simulink model "VITM_OL_Harness"  (R2017b)
settings: Solver=ode4  StartTime=0.0  StopTime=sim_time  FixedStep=0.01  RelTol=1e-3  EnableMultiTasking=on
settings Model: Creator=favv5g  LastModifiedBy=nctzv8
settings DataIOCC: LimitDataPoints=on
settings OptimizationCC: LifeSpan=inf
settings DebuggingCC: MultiTaskRateTransMsg=warning  SingleTaskRateTransMsg=warning  AllowSymbolicDim=off  SFUnexpectedBacktrackingDiag=warning  SFNoUnconditionalDefaultTransitionDiag=warning  SFExecutionAtInitializationDiag=none
settings HardwareCC: ProdBitPerPointer=32  ProdBitPerSizeT=32  ProdBitPerPtrDiffT=32  ProdLargestAtomicInteger=Long  ProdLargestAtomicFloat=Double  ProdEndianess=BigEndian  ProdWordSize=32  ProdHWDeviceType=Freescale->32-bit PowerPC
settings ModelReferenceCC: PropagateSignalLabelsOutOfModel=off
settings CodeAppCC: StateflowObjectComments=on
settings GRTTargetCC: TargetLangStandard=C89/C90 (ANSI)
settings ConfigComp: CovMetricSettings=dw  CovHtmlReporting=on  CovSaveCumulativeToWorkspaceVar=on  CovSaveSingleToWorkspaceVar=on  CovExternalEMLEnable=off

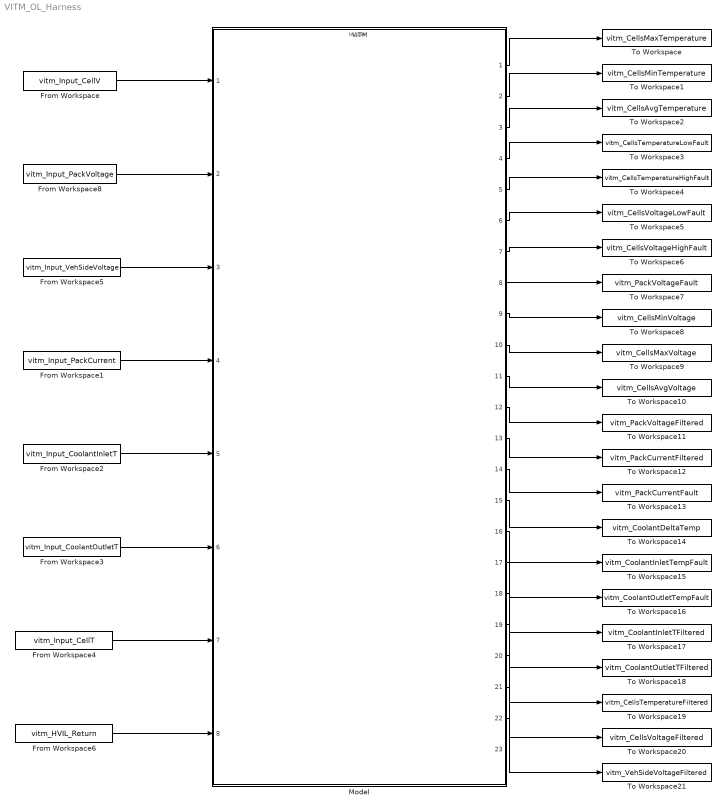
== system VITM_OL_Harness ==
  From Workspace : FromWorkspace  VariableName=vitm_Input_CellV  SampleTime=0
  From Workspace1 : FromWorkspace  VariableName=vitm_Input_PackCurrent  SampleTime=0
  From Workspace2 : FromWorkspace  VariableName=vitm_Input_CoolantInletT  SampleTime=0
  From Workspace3 : FromWorkspace  VariableName=vitm_Input_CoolantOutletT  SampleTime=0
  From Workspace4 : FromWorkspace  VariableName=vitm_Input_CellT  SampleTime=0
  From Workspace5 : FromWorkspace  VariableName=vitm_Input_VehSideVoltage  SampleTime=0
  From Workspace6 : FromWorkspace  VariableName=vitm_HVIL_Return  SampleTime=0
  From Workspace8 : FromWorkspace  VariableName=vitm_Input_PackVoltage  SampleTime=0
  Model : ModelReference  ModelNameDialog=VITM.slx  SimulationMode=Normal  ModelReferenceVersion=1.124  TriggerPortName=Trigger  TriggerPortTriggerType=function-call  TriggerPortStatesWhenEnabling=held
  To Workspace : ToWorkspace  VariableName=vitm_CellsMaxTemperature  SaveFormat=Timeseries  SampleTime=-1
  To Workspace1 : ToWorkspace  VariableName=vitm_CellsMinTemperature  SaveFormat=Timeseries  SampleTime=-1
  To Workspace10 : ToWorkspace  VariableName=vitm_CellsAvgVoltage  SaveFormat=Timeseries  SampleTime=-1
  To Workspace11 : ToWorkspace  VariableName=vitm_PackVoltageFiltered  SaveFormat=Timeseries  SampleTime=-1
  To Workspace12 : ToWorkspace  VariableName=vitm_PackCurrentFiltered  SaveFormat=Timeseries  SampleTime=-1
  To Workspace13 : ToWorkspace  VariableName=vitm_PackCurrentFault  SaveFormat=Timeseries  SampleTime=-1
  To Workspace14 : ToWorkspace  VariableName=vitm_CoolantDeltaTemp  SaveFormat=Timeseries  SampleTime=-1
  To Workspace15 : ToWorkspace  VariableName=vitm_CoolantInletTempFault  SaveFormat=Timeseries  SampleTime=-1
  To Workspace16 : ToWorkspace  VariableName=vitm_CoolantOutletTempFault  SaveFormat=Timeseries  SampleTime=-1
  To Workspace17 : ToWorkspace  VariableName=vitm_CoolantInletTFiltered  SaveFormat=Timeseries  SampleTime=-1
  To Workspace18 : ToWorkspace  VariableName=vitm_CoolantOutletTFiltered  SaveFormat=Timeseries  SampleTime=-1
  To Workspace19 : ToWorkspace  VariableName=vitm_CellsTemperatureFiltered  SaveFormat=Timeseries  SampleTime=-1
  To Workspace2 : ToWorkspace  VariableName=vitm_CellsAvgTemperature  SaveFormat=Timeseries  SampleTime=-1
  To Workspace20 : ToWorkspace  VariableName=vitm_CellsVoltageFiltered  SaveFormat=Timeseries  SampleTime=-1
  To Workspace21 : ToWorkspace  VariableName=vitm_VehSideVoltageFiltered  SaveFormat=Timeseries  SampleTime=-1
  To Workspace3 : ToWorkspace  VariableName=vitm_CellsTemperatureLowFault  SaveFormat=Timeseries  SampleTime=-1
  To Workspace4 : ToWorkspace  VariableName=vitm_CellsTemperatureHighFault  SaveFormat=Timeseries  SampleTime=-1
  To Workspace5 : ToWorkspace  VariableName=vitm_CellsVoltageLowFault  SaveFormat=Timeseries  SampleTime=-1
  To Workspace6 : ToWorkspace  VariableName=vitm_CellsVoltageHighFault  SaveFormat=Timeseries  SampleTime=-1
  To Workspace7 : ToWorkspace  VariableName=vitm_PackVoltageFault  SaveFormat=Timeseries  SampleTime=-1
  To Workspace8 : ToWorkspace  VariableName=vitm_CellsMinVoltage  SaveFormat=Timeseries  SampleTime=-1
  To Workspace9 : ToWorkspace  VariableName=vitm_CellsMaxVoltage  SaveFormat=Timeseries  SampleTime=-1
  wires:
  From Workspace/1 -> Model/1
  Model/1 -> To Workspace/1
  Model/2 -> To Workspace1/1
  Model/3 -> To Workspace2/1
  Model/4 -> To Workspace3/1
  Model/5 -> To Workspace4/1
  Model/6 -> To Workspace5/1
  Model/7 -> To Workspace6/1
  Model/8 -> To Workspace7/1
  Model/9 -> To Workspace8/1
  Model/10 -> To Workspace9/1
  Model/11 -> To Workspace10/1
  Model/12 -> To Workspace11/1
  Model/13 -> To Workspace12/1
  Model/14 -> To Workspace13/1
  Model/15 -> To Workspace14/1
  Model/16 -> To Workspace15/1
  Model/17 -> To Workspace16/1
  Model/18 -> To Workspace17/1
  Model/19 -> To Workspace18/1
  Model/20 -> To Workspace19/1
  Model/21 -> To Workspace20/1
  From Workspace4/1 -> Model/7
  From Workspace3/1 -> Model/6
  From Workspace2/1 -> Model/5
  From Workspace1/1 -> Model/4
  From Workspace5/1 -> Model/3
  From Workspace8/1 -> Model/2
  Model/22 -> To Workspace21/1
  From Workspace6/1 -> Model/8
